simulink model "DSOGI_PLL_ThreePhase"  (R2022b)
settings: Solver=FixedStepDiscrete  StartTime=0.0  StopTime=4  FixedStep=1e-6  RelTol=1e-3
libraries: spspowerguiLib x1
settings Model: Creator=XIAO  LastModifiedBy=XIAO
settings SolverCC: AutoInsertRateTranBlk=on
settings DataIOCC: ReturnWorkspaceOutputs=off

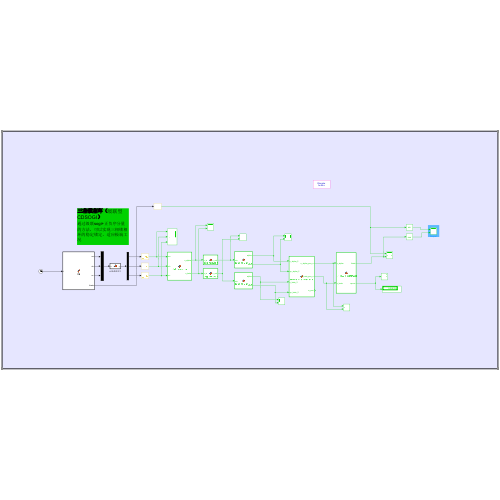
[thumbnail: Simulink's stored preview of the top-level diagram]
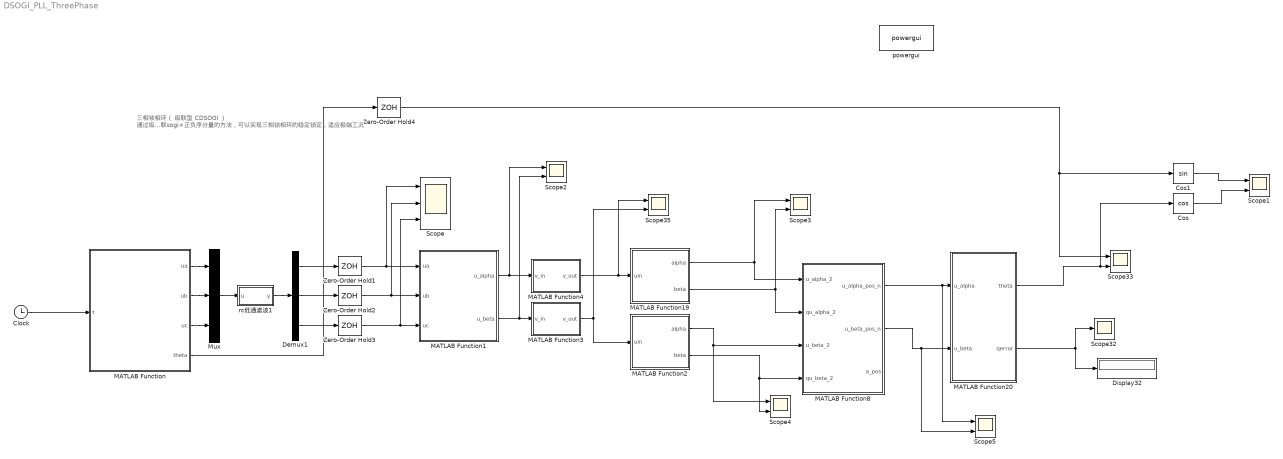
== system DSOGI_PLL_ThreePhase ==
  note: 三相锁相环（ 级联型 CDSOGI ）
      | 通过级联sogi+正负序分量的方法，可以实现三相锁相环的稳定锁定，适应极端工况
  Clock : Clock
  Cos : Trigonometry  Operator=cos
  Cos1 : Trigonometry
  Demux1 : Demux  Outputs=3
  Display32 : Display
  MATLAB Function : MATLAB Function  TreatAsAtomicUnit=on
  MATLAB Function1 : MATLAB Function  TreatAsAtomicUnit=on
  MATLAB Function19 : MATLAB Function  TreatAsAtomicUnit=on
  MATLAB Function2 : MATLAB Function  TreatAsAtomicUnit=on
  MATLAB Function20 : MATLAB Function  TreatAsAtomicUnit=on
  MATLAB Function3 : MATLAB Function  TreatAsAtomicUnit=on
  MATLAB Function4 : MATLAB Function  TreatAsAtomicUnit=on
  MATLAB Function8 : MATLAB Function  TreatAsAtomicUnit=on
  Mux : Mux  Inputs=3
  Scope : Scope  NumInputPorts=3
  Scope{1..5,33,35} (7 alike) : Scope  NumInputPorts=2
  Scope32 : Scope
  Zero-Order Hold{1..4} (4 alike) : ZeroOrderHold  SampleTime=5e-5
  powergui : spspowerguiLib/powergui  Priority=1  SimulationMode=Discrete  SampleTime=1e-6  frequency=60  Iterations=50  frequencyindice=60  Pbase=100e6  ErrMax=1e-4  UnitsV=kV  UnitsW=MW  buscounter=0  FunctionMessages=off  echomessages=off  EnableUseOfTLC=off  CurrentSourceSwitches=off  DisableSnubberDevices=off  DisableRonSwitches=off  DisableVfSwitches=off  DisplayEquations=off  AutomaticDiscreteSolvers=off  SolverType=Tustin/Backward Euler (TBE)  Interpol=off  ExternalGateDelay=off  methode=off  Ts=100  x0status=blocks  SPID=on  SwTol=0  HookPort=off  NonlinearTolerance=1e-4  nMaxIteration=100  ContinueOnMaxIteration=off  RestoreLinks=warning  ResistiveCurrentMeasurement=off  Frange=[0:2:500]  Ylog=off  Xlog=on  ShowGrid=off  save=off  variable=ZData  structure=0  ZoomFFT=off  StartTime=0.0  cycles=1  DisplayStyle=1  fundamental=60  FreqAxis=off  MaxFrequency=1000  frequencyindicesteady=1  RmsSteady=1  display=off
  rc低通滤波1 : MATLAB Function  TreatAsAtomicUnit=on
  wires:
  Clock/1 -> MATLAB Function/1(t)
  MATLAB Function20/1(theta) -> Cos/1, Scope33/2
  MATLAB Function20/2(qerror) -> Scope32/1, Display32/1
  MATLAB Function/4(theta) -> Zero-Order Hold4/1
  Zero-Order Hold2/1 -> Scope/2, MATLAB Function1/2(ub)
  Zero-Order Hold1/1 -> Scope/1, MATLAB Function1/1(ua)
  Zero-Order Hold3/1 -> Scope/3, MATLAB Function1/3(uc)
  MATLAB Function19/1(alpha) -> Scope3/1, MATLAB Function8/1(u_alpha_2)
  MATLAB Function19/2(beta) -> Scope3/2, MATLAB Function8/2(qu_alpha_2)
  MATLAB Function2/1(alpha) -> Scope4/1, MATLAB Function8/3(u_beta_2)
  MATLAB Function2/2(beta) -> Scope4/2, MATLAB Function8/4(qu_beta_2)
  MATLAB Function8/1(u_alpha_pos_n) -> Scope5/1, MATLAB Function20/1(u_alpha)
  Zero-Order Hold4/1 -> Scope33/1, Cos1/1
  MATLAB Function1/1(u_alpha) -> MATLAB Function4/1(v_in), Scope2/1
  MATLAB Function1/2(u_beta) -> MATLAB Function3/1(v_in), Scope2/2
  MATLAB Function4/1(v_out) -> Scope35/1, MATLAB Function19/1(uin)
  MATLAB Function3/1(v_out) -> MATLAB Function2/1(uin), Scope35/2
  Cos1/1 -> Scope1/1
  Cos/1 -> Scope1/2
  MATLAB Function8/2(u_beta_pos_n) -> Scope5/2, MATLAB Function20/2(u_beta)
  MATLAB Function/2(ub) -> Mux/2
  MATLAB Function/1(ua) -> Mux/1
  MATLAB Function/3(uc) -> Mux/3
  Mux/1 -> rc低通滤波1/1(u)
  rc低通滤波1/1(y) -> Demux1/1
  Demux1/2 -> Zero-Order Hold2/1
  Demux1/3 -> Zero-Order Hold3/1
  Demux1/1 -> Zero-Order Hold1/1

== matlab function DSOGI_PLL_ThreePhase/MATLAB Function ==
  data: ua output; t input; ub output; uc output; theta output
function [ua, ub, uc, theta] = fcn(t)
% 纯粹故障源进阶版：三阶段极端非理想三相电网生成器（含高阶杂乱谐波与接地过电压）
% 工况1：0-1s 理想对称电网
% 工况2：1-2s 相位差最大偏移5° + 原极端幅值不对称 + 3/5/7/9/11次谐波 + 直流偏置
% 工况3：2-3s A相完全接地故障（B、C相符合线电压抬升的实际物理逻辑）

%% ====================== 常量与持久化变量 ======================
persistent t_prev phi_dynamic first_run U_amp
persistent t_switch1 t_switch2
persistent harsh_amp_a harsh_amp_b harsh_amp_c
persistent harsh_phase_a harsh_phase_b harsh_phase_c
persistent h3_ratio h5_ratio h7_ratio h9_ratio h11_ratio
persistent dc_phase2_a dc_phase2_b dc_phase2_c dc_phase3

if isempty(first_run)
    t_prev = 0;
    phi_dynamic = 0; % 基波连续参考相位（rad）
    
    t_switch1 = 1.0;
    t_switch2 = 2.0;
    
    U_rms = 32;
    U_amp = U_rms * sqrt(2); 
    
    % --- 工况2：极端幅值不对称设定 ---
    harsh_amp_a = 1.0; harsh_amp_b = 0.8; harsh_amp_c = 0.6;
    
    % --- 工况2/3：非对称相位差设定（最大偏移5°） ---
    harsh_phase_a = deg2rad(0);
    harsh_phase_b = deg2rad(-122.5);  % B相比理想滞后2.5°
    harsh_phase_c = deg2rad(122.5);   % C相比理想超前2.5°
    
    % --- 谐波参数库（新增9次、11次高频杂乱谐波） ---
    h3_ratio  = 0.05;   % 3次零序谐波（5%）
    h5_ratio  = 0.04;   % 5次负序谐波（4%）
    h7_ratio  = 0.03;   % 7次正序谐波（3%）
    h9_ratio  = 0.02;   % 9次零序杂乱谐波（2%）
    h11_ratio = 0.015;  % 11次负序杂乱谐波（1.5%）
    
    % --- 直流偏置参数 ---
    dc_phase2_a = 5; dc_phase2_b = 6; dc_phase2_c = 7; 
    dc_phase3 = 6;
    
    first_run = false;
end

%% ====================== 1. 物理连续时间积分 ======================
dt = t - t_prev;
if dt <= 0, dt = 5e-5; end

% --- 频率步进故障 ---
if t < t_switch1
    f_current = 50; 
else
    f_current = 45; % 1s后频率跌落至45Hz
end
phi_dynamic = phi_dynamic + 2 * pi * f_current * dt;
t_prev = t;

%% ====================== 2. 分阶段合成三相电压 ======================
if t < t_switch1
    %% =============================================================
    % 【工况1】：0-1s 理想对称电网
    %% =============================================================
    ua = U_amp * sin(phi_dynamic + deg2rad(0));
    ub = U_amp * sin(phi_dynamic + deg2rad(-120));
    uc = U_amp * sin(phi_dynamic + deg2rad(120));
    
elseif t < t_switch2
    %% =============================================================
    % 【工况2】：1-2s 极端复合不平衡与多重高次谐波污染（杂乱网络）
    %  - 谐波成分：叠加3、5、7、9、11次全谱系干扰
    %% =============================================================
    % 基波生成
    ua_base = harsh_amp_a * U_amp * sin(phi_dynamic + harsh_phase_a);
    ub_base = harsh_amp_b * U_amp * sin(phi_dynamic + harsh_phase_b);
    uc_base = harsh_amp_c * U_amp * sin(phi_dynamic + harsh_phase_c);
    
    % 谐波矩阵计算
    h3 = h3_ratio * U_amp * sin(3 * phi_dynamic);
    h5_a = h5_ratio * U_amp * sin(5 * phi_dynamic);
    h5_b = h5_ratio * U_amp * sin(5 * phi_dynamic + 2*pi/3);
    h5_c = h5_ratio * U_amp * sin(5 * phi_dynamic - 2*pi/3);
    h7_a = h7_ratio * U_amp * sin(7 * phi_dynamic);
    h7_b = h7_ratio * U_amp * sin(7 * phi_dynamic - 2*pi/3);
    h7_c = h7_ratio * U_amp * sin(7 * phi_dynamic + 2*pi/3);
    
    % 新增：9次（零序，同相位）与11次（负序，相位反转）
    h9  = h9_ratio * U_amp * sin(9 * phi_dynamic);
    h11_a = h11_ratio * U_amp * sin(11 * phi_dynamic);
    h11_b = h11_ratio * U_amp * sin(11 * phi_dynamic + 2*pi/3);
    h11_c = h11_ratio * U_amp * sin(11 * phi_dynamic - 2*pi/3);
    
    % 复合全信号输出
    ua = ua_base + h3 + h5_a + h7_a + h9 + h11_a + dc_phase2_a;
    ub = ub_base + h3 + h5_b + h7_b + h9 + h11_b + dc_phase2_b;
    uc = uc_base + h3 + h5_c + h7_c + h9 + h11_c + dc_phase2_c;
    
else
    %% =============================================================
    % 【工况3】：2-3s A相完全接地短路（引入物理过电压逻辑）
    %  - A相：短路接地归零。
    %  - B/C相幅值变化逻辑：由于A相接地，非故障相对地电压强行抬升 sqrt(3) 倍
    %  - 谐波与直流：A相谐波消失；B、C相继续承受3、5、7、9、11次严重谐波冲击
    %% =============================================================
    ua = 0.0; % A相完全接地归零
    
    % 关键修改：非故障相基波幅值乘以 sqrt(3)，模拟金属性单相接地后的线电压抬升
    ub_base = (harsh_amp_b * sqrt(3)) * U_amp * sin(phi_dynamic + harsh_phase_b);
    uc_base = (harsh_amp_c * sqrt(3)) * U_amp * sin(phi_dynamic + harsh_phase_c);
    
    % B、C相残留的杂乱多重谐波
    h3 = h3_ratio * U_amp * sin(3 * phi_dynamic);
    h5_b = h5_ratio * U_amp * sin(5 * phi_dynamic + 2*pi/3);
    h5_c = h5_ratio * U_amp * sin(5 * phi_dynamic - 2*pi/3);
    h7_b = h7_ratio * U_amp * sin(7 * phi_dynamic - 2*pi/3);
    h7_c = h7_ratio * U_amp * sin(7 * phi_dynamic + 2*pi/3);
    
    h9  = h9_ratio * U_amp * sin(9 * phi_dynamic);
    h11_b = h11_ratio * U_amp * sin(11 * phi_dynamic + 2*pi/3);
    h11_c = h11_ratio * U_amp * sin(11 * phi_dynamic - 2*pi/3);
    
    % 合成最终的故障过电压信号
    ub = ub_base + h3 + h5_b + h7_b + h9 + h11_b + dc_phase3;
    uc = uc_base + h3 + h5_c + h7_c + h9 + h11_c + dc_phase3;
end

%% ====================== 3. 输出纯粹的 A 相零点参考角 ======================
theta = mod(phi_dynamic, 2*pi);

end

== matlab function DSOGI_PLL_ThreePhase/MATLAB Function1 ==
  data: ua input; u_alpha output; ub input; uc input; u_beta output
function [u_alpha, u_beta] = clark_transform(ua, ub, uc)
% 三相静止坐标系(abc)到两相静止坐标系(αβ)的等幅值变换
% 电力电子控制行业标准实现，与SRF-PLL、SVPWM等算法完全兼容
% 输入：ua, ub, uc = 三相相电压（或电流）瞬时值
% 输出：u_alpha, u_beta = 两相静止坐标系α、β轴分量

%% 预计算常数（仅首次调用计算一次，提高效率）
persistent SQRT3_OVER_2 COEFF_2_OVER_3
if isempty(SQRT3_OVER_2)
    SQRT3_OVER_2 = sqrt(3) / 2;  % √3/2 ≈ 0.8660254
    COEFF_2_OVER_3 = 2.0 / 3.0;  % 2/3 ≈ 0.6666667
end

%% 等幅值克拉克变换核心公式
u_alpha = COEFF_2_OVER_3 * (ua - 0.5*ub - 0.5*uc);
u_beta  = COEFF_2_OVER_3 * (SQRT3_OVER_2*ub - SQRT3_OVER_2*uc);

end

== matlab function DSOGI_PLL_ThreePhase/MATLAB Function2 ==
  settings: updateMethod=DISCRETE
  data: uin input; alpha output; beta output
function [alpha, beta] = SOGI_FLL_20kHz(uin)
% 严格对应你的 m 文件：20kHz 双线性 PI-FLL
% 输入：uin   单相电压
% 输出：alpha 同相输出 uα = x2
%      beta  正交输出 uβ = omega0*x3

%% 固定参数（和你的m文件完全一致）
dt = 5e-5;
K  = 1.414;
K1 = 0.25;
gamma_p =30;
gamma_i =500;
w_max = 2*pi*60;
w_min = 2*pi*40;

%% 状态持久化
persistent x1_prev x2_prev x3_prev omega0_prev U_prev integral_f first_run;
if isempty(first_run)
    x1_prev = 0;
    x2_prev = 0;
    x3_prev = 0;
    omega0_prev = 2*pi*50;
    U_prev = uin;
    integral_f = 0;
    first_run = false;
end

%% 1. 当前输入
U_curr = uin;
omega0_prev_local = omega0_prev;

%% 2. 频率预畸变
omega_pre = (2/dt) * tan(omega0_prev_local * dt / 2);

%% 3. 状态矩阵 A, B
A_mat = [
    -K1*omega_pre, -K1*omega_pre, 0;
    -K*omega_pre,  -K*omega_pre,  -omega_pre^2;
    0,              1,              0
];
B_mat = [
    K1*omega_pre;
    K*omega_pre;
    0
];

%% 4. 双线性变换
I_mat = eye(3);
M1 = I_mat - (dt/2)*A_mat;
M2 = I_mat + (dt/2)*A_mat;
U_avg = U_curr + U_prev;

x_prev_vec = [x1_prev; x2_prev; x3_prev];
x_curr_vec = M1 \ (M2 * x_prev_vec + (dt/2)*B_mat * U_avg);

x1_curr = x_curr_vec(1);
x2_curr = x_curr_vec(2);
x3_curr = x_curr_vec(3);

%% 5. PI-FLL 频率环
deltaU = U_curr - x1_curr - x2_curr;
deltaU_prime_val = omega0_prev_local * x3_curr;
epsilon_f = deltaU * deltaU_prime_val;

integral_f = integral_f + epsilon_f * dt;
domega0dt = -gamma_p * epsilon_f - gamma_i * integral_f;
omega0_curr = omega0_prev_local + dt * domega0dt;

% 频率限幅
omega0_curr = max(min(omega0_curr, w_max), w_min);

%% 6. 输出 alpha beta
alpha = x2_curr;
beta  = omega0_curr * x3_curr;

%% 7. 更新状态
x1_prev = x1_curr;
x2_prev = x2_curr;
x3_prev = x3_curr;
omega0_prev = omega0_curr;
U_prev = U_curr;

end

== matlab function DSOGI_PLL_ThreePhase/MATLAB Function4 ==
  data: v_in input; v_out output

function v_out = sogi_qsg_module_fixed(v_in)

% 固定频率版：无频率反馈 SOGI-QSG 正交信号发生器

% 额定频率：50Hz，采样周期：50us(20kHz)

% 修复MATLAB Coder变量未定义错误

% 所有编译期常量移到persistent块外，确保所有执行路径可见

%% 1. 编译期常量（代码生成时直接替换为数值，不占用运行时间）

Ts = 50e-6; % 20kHz采样周期

w_nominal = 2*pi*50; % 固定50Hz额定角频率

k = 2.0; % 保留原增益优化值

phi_comp = 34*pi/180;% 保留原35°相位补偿


% 预计算所有常数系数（代码生成时自动计算，运行时无开销）

A = 2 / Ts;

det = A^2 + A*k*w_nominal + w_nominal^2;

b0 = k*w_nominal*A;

cos_phi = cos(phi_comp);

sin_phi = sin(phi_comp);

%% 2. 仅状态变量使用persistent

persistent initialized x1 x2

if isempty(initialized)

x1 = 0.0;

x2 = 0.0;

initialized = 1;

end

%% 3. SOGI核心计算（完全不变）

v_prime = (b0*v_in + (A^2 - w_nominal^2)*x1 - 2*w_nominal*A*x2) / det;

qv_prime = (w_nominal*A*v_in + 2*w_nominal*A*x1 + (A^2 - k*w_nominal*A)*x2) / det;

%% 4. 主动相位补偿（完全不变）

v_out = v_prime*cos_phi - qv_prime*sin_phi;

%% 5. 更新状态变量（完全不变）

x1 = v_prime;

x2 = qv_prime;

end

== matlab function DSOGI_PLL_ThreePhase/MATLAB Function3 ==
  data: v_in input; v_out output


function v_out = sogi_qsg_module_fixed(v_in)

% 固定频率版：无频率反馈 SOGI-QSG 正交信号发生器

% 额定频率：50Hz，采样周期：50us(20kHz)

% 修复MATLAB Coder变量未定义错误

% 所有编译期常量移到persistent块外，确保所有执行路径可见

%% 1. 编译期常量（代码生成时直接替换为数值，不占用运行时间）

Ts = 50e-6; % 20kHz采样周期

w_nominal = 2*pi*50; % 固定50Hz额定角频率

k = 2.0; % 保留原增益优化值

phi_comp = 34*pi/180;% 保留原35°相位补偿


% 预计算所有常数系数（代码生成时自动计算，运行时无开销）

A = 2 / Ts;

det = A^2 + A*k*w_nominal + w_nominal^2;

b0 = k*w_nominal*A;

cos_phi = cos(phi_comp);

sin_phi = sin(phi_comp);

%% 2. 仅状态变量使用persistent

persistent initialized x1 x2

if isempty(initialized)

x1 = 0.0;

x2 = 0.0;

initialized = 1;

end

%% 3. SOGI核心计算（完全不变）

v_prime = (b0*v_in + (A^2 - w_nominal^2)*x1 - 2*w_nominal*A*x2) / det;

qv_prime = (w_nominal*A*v_in + 2*w_nominal*A*x1 + (A^2 - k*w_nominal*A)*x2) / det;

%% 4. 主动相位补偿（完全不变）

v_out = v_prime*cos_phi - qv_prime*sin_phi;

%% 5. 更新状态变量（完全不变）

x1 = v_prime;

x2 = qv_prime;

end

== matlab function DSOGI_PLL_ThreePhase/rc低通滤波1 ==
  data: u input; y output
function y = fcn(u)
%#codegen
% 三相专用一阶RC低通滤波（Simulink Coder 100%兼容版）
% 适配：三相3×1向量输入，Ts=1e-6s，fc=4.7kHz
% 输入：u - 三相原始信号 [Ua; Ub; Uc] (3×1)
% 输出：y - 三相滤波后信号 [Ua_filt; Ub_filt; Uc_filt] (3×1)
% 作者：Power Bell
% 日期：2026-05-20

% 持久化状态变量（仅保存上一时刻三相输出）
persistent y_prev;

% ---------------- 关键修复1：显式声明所有变量尺寸 ----------------
% 强制y_prev为固定3×1尺寸（禁止动态数组）
coder.varsize('y_prev', [3 1], [0 0]);
% 显式声明输出y为3×1尺寸，彻底解决Simulink无法推断输出大小的问题
y = zeros(3, 1);
% ----------------------------------------------------------------

% ---------------- 预计算常量（MATLAB Coder自动优化为编译时常量） ----------------
% 精确计算值：alpha = exp(-1e-6/(1/(2*pi*4700))) = 0.970903023515853
% 精确计算值：beta = 1 - alpha = 0.029096976484147
alpha = 0.970903023515853;
beta  = 0.029096976484147;
% ----------------------------------------------------------------

% 初始化状态（仅第一次调用执行）
if isempty(y_prev)
    y_prev = zeros(3, 1);
end

% 三相独立滤波差分方程（向量化运算，最高效率）
y = alpha * y_prev + beta * u;

% 更新状态变量
y_prev = y;

end

== matlab function DSOGI_PLL_ThreePhase/MATLAB Function8 ==
  data: u_alpha_2 input; u_alpha_pos_n output; qu_alpha_2 input; u_beta_2 input; qu_beta_2 input; u_beta_pos_n output; a_pos output
function [u_alpha_pos_n, u_beta_pos_n, a_pos] = positive_sequence_calc(u_alpha_2, qu_alpha_2, u_beta_2, qu_beta_2)
% 论文级联型CDSOGI的正序分量计算及归一化模块
% 输入：
%   u_alpha_2  = 后级α轴SOGI的同相输出 uα''
%   qu_alpha_2 = 后级α轴SOGI的正交输出 quα''
%   u_beta_2   = 后级β轴SOGI的同相输出 uβ''
%   qu_beta_2  = 后级β轴SOGI的正交输出 quβ''
% 输出：
%   u_alpha_pos_n = 归一化后的正序分量α轴 (单位化向量)
%   u_beta_pos_n  = 归一化后的正序分量β轴 (单位化向量)
%   a_pos         = 正序分量的实际幅值（可选输出，方便观测）

%% 1. 正序分量核心计算（与图中逻辑100%一致）
u_alpha_pos = 0.5 * u_alpha_2 - 0.5 * qu_beta_2;
u_beta_pos  = 0.5 * qu_alpha_2 + 0.5 * u_beta_2;

%% 2. 计算正序分量的瞬时幅值
% 使用合成向量模长公式：A = sqrt(alpha^2 + beta^2)
a_pos = sqrt(u_alpha_pos^2 + u_beta_pos^2);

%% 3. 归一化处理（带防除零保护）
% eps 是 MATLAB 内置极小值（约 2.22e-16），防止分母为 0 导致 NaN 错误
u_alpha_pos_n = u_alpha_pos / (a_pos + eps);
u_beta_pos_n  = u_beta_pos / (a_pos + eps);

end

== matlab function DSOGI_PLL_ThreePhase/MATLAB Function19 ==
  settings: updateMethod=DISCRETE
  data: uin input; alpha output; beta output
function [alpha, beta] = SOGI_FLL_20kHz(uin)
% 20kHz 双线性 PI-FLL（已新增角频率 w_out 输出端口）
% 输入：uin       单相电压
% 输出：alpha     同相输出 uα = x2
%      beta      正交输出 uβ = omega0*x3
%      freq_out  跟踪到的电网频率（单位：Hz）
%      w_out     跟踪到的电网角频率（单位：rad/s）-> 新增端口

%% 固定参数
dt = 5e-5;
K  = 1.414;
K1 = 0.25;
gamma_p = 30;
gamma_i = 500;
w_max = 2*pi*60;
w_min = 2*pi*40;

%% 状态持久化
persistent x1_prev x2_prev x3_prev omega0_prev U_prev integral_f first_run;
if isempty(first_run)
    x1_prev = 0;
    x2_prev = 0;
    x3_prev = 0;
    omega0_prev = 2*pi*50;
    U_prev = uin;
    integral_f = 0;
    first_run = false;
end

%% 1. 当前输入
U_curr = uin;
omega0_prev_local = omega0_prev;

%% 2. 频率预畸变
omega_pre = (2/dt) * tan(omega0_prev_local * dt / 2);

%% 3. 状态矩阵 A, B
A_mat = [
    -K1*omega_pre, -K1*omega_pre, 0;
    -K*omega_pre,  -K*omega_pre,  -omega_pre^2;
    0,              1,              0
];
B_mat = [
    K1*omega_pre;
    K*omega_pre;
    0
];

%% 4. 双线性变换
I_mat = eye(3);
M1 = I_mat - (dt/2)*A_mat;
M2 = I_mat + (dt/2)*A_mat;
U_avg = U_curr + U_prev;
x_prev_vec = [x1_prev; x2_prev; x3_prev];
x_curr_vec = M1 \ (M2 * x_prev_vec + (dt/2)*B_mat * U_avg);
x1_curr = x_curr_vec(1);
x2_curr = x_curr_vec(2);
x3_curr = x_curr_vec(3);

%% 5. PI-FLL 频率环
deltaU = U_curr - x1_curr - x2_curr;
deltaU_prime_val = omega0_prev_local * x3_curr;
epsilon_f = deltaU * deltaU_prime_val;
integral_f = integral_f + epsilon_f * dt;
domega0dt = -gamma_p * epsilon_f - gamma_i * integral_f;
omega0_curr = omega0_prev_local + dt * domega0dt;

% 频率限幅
omega0_curr = max(min(omega0_curr, w_max), w_min);

%% 6. 输出分配
alpha = x2_curr;
beta  = omega0_curr * x3_curr;

%% 7. 更新状态
x1_prev = x1_curr;
x2_prev = x2_curr;
x3_prev = x3_curr;
omega0_prev = omega0_curr;
U_prev = U_curr;
end

== matlab function DSOGI_PLL_ThreePhase/MATLAB Function20 ==
  data: u_alpha input; theta output; u_beta input; qerror output
function [theta, qerror] = SRF_PLL_Feedforward(u_alpha, u_beta)
    % 彻底重构版：去前馈 + 固定高动态响应 PLL
    
    %% ===================== 1. 固定高动态参数 =====================
    Ts = 5e-5;               
    
    % 固定高增益参数：不再搞动态切换，防止阈值误触发
    % Kp = 200 能够提供足够强劲的暂态追赶速度
    % Ki = 7000 保证稳态下无静差，并且能快速吃掉 SOGI 传过来的任何残余滞后
    kp_pll = 200;   
    ki_pll = 7000;  
    
    % 放弃波动剧烈的 FLL 前馈，改用 50Hz 固定的额定基准角频率
    omega_rated = 2 * pi * 50; 
    
    %% ===================== 2. 持久变量 =====================
    persistent theta_prev
    persistent integral_pll
    
    if isempty(theta_prev)
        theta_prev = 0;
        integral_pll = 0;
    end
    
    %% ===================== 3. Park 变换 =====================
    cos_theta = cos(theta_prev);
    sin_theta = sin(theta_prev);
    
    u_d =  u_alpha * cos_theta + u_beta * sin_theta;
    u_q = -u_alpha * sin_theta + u_beta * cos_theta;
    
    qerror = u_q;  
    
    %% ===================== 4. 标准 PI 控制器（不带 FLL 前馈干扰） =====================
    integral_pll = integral_pll + qerror * Ts;          
    
    % 使用固定的额定 50Hz 作为前馈基准，PI 控制器完全闭环自主调节
    omega_pll = omega_rated + (kp_pll * qerror + ki_pll * integral_pll); 
    
    %% ===================== 5. 积分生成相位 =====================
    theta = theta_prev + omega_pll * Ts;
    
    %% 相位归一化
    theta = mod(theta, 2*pi);
    if theta < 0
        theta = theta + 2*pi;
    end
    
    %% ===================== 6. 更新状态 =====================
    theta_prev = theta;
end
